simulink model "Solar_panel"  (R2024a)
settings: Solver=VariableStepAuto  StartTime=0.0  StopTime=1000  RelTol=1e-3
libraries: ee_lib x36, fl_lib x5, nesl_utility x4, simulink x1
settings Model: SimulationMode=accelerator  Creator=glenn  LastModifiedBy=glenn

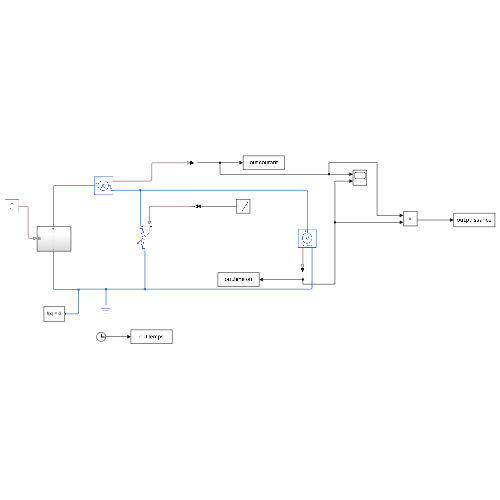
[thumbnail: Simulink's stored preview of the top-level diagram]
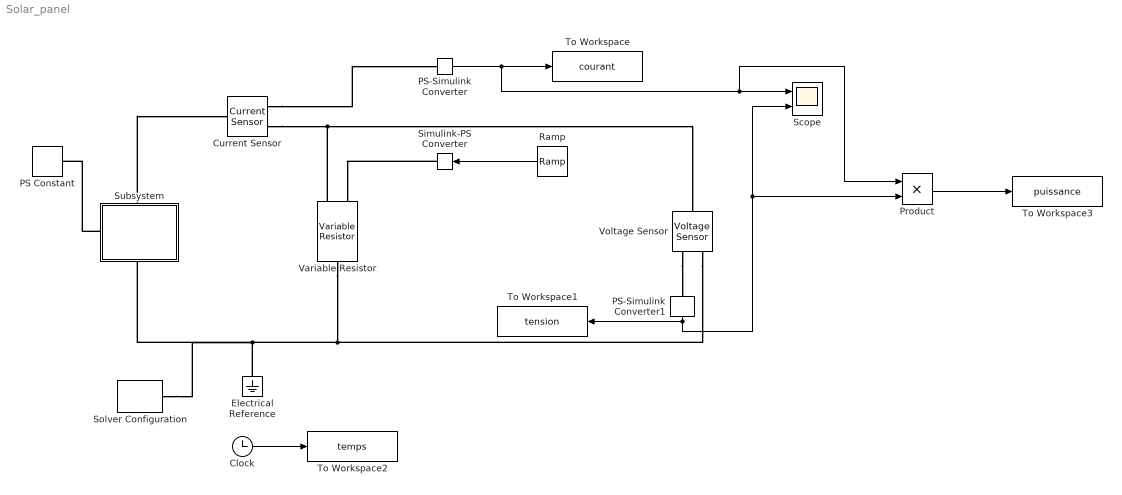
== system Solar_panel ==
  Clock : Clock
  Current Sensor : fl_lib/Electrical/Electrical Sensors/Current Sensor
  Electrical Reference : fl_lib/Electrical/Electrical Elements/Electrical Reference
  PS Constant : fl_lib/Physical Signals/Sources/PS Constant  constant=1000
  PS-Simulink Converter : nesl_utility/PS-Simulink Converter  PhysicalDomain=network_engine_domain  SubClassName=ps_output  LeftPortType=input  RightPortType=output  PseudoPeriodic=off  Frequencies=[]  VectorFormat=inherit  Unit=inherit  AffineConversion=off
  PS-Simulink Converter1 : nesl_utility/PS-Simulink Converter  PhysicalDomain=network_engine_domain  SubClassName=ps_output  LeftPortType=input  RightPortType=output  PseudoPeriodic=off  Frequencies=[]  VectorFormat=inherit  Unit=inherit  AffineConversion=off
  Product : Product
  Ramp : simulink/Sources/Ramp  slope=1  start=0  InitialOutput=0
  Scope : Scope  NumInputPorts=2
  Simulink-PS Converter : nesl_utility/Simulink-PS Converter  PhysicalDomain=network_engine_domain  SubClassName=ps_input  LeftPortType=input  RightPortType=output  PseudoPeriodic=off  Frequencies=[]  NoiseDistribution=none  NoiseParameters=[]  Unit=1  AffineConversion=off  FilteringAndDerivatives=provide  SimscapeFilterOrder=1  InputFilterTimeConstant=0.001  UdotUserProvided=0
  Solver Configuration : nesl_utility/Solver Configuration  PhysicalDomain=network_engine_domain  SubClassName=solver  LeftPortType=input  RightPortType=generic  Tones=[]  Harmonics=[]  SimulateNoise=off  Profile=off  UseLocalSampling=off  EnableSwitchedLinearOptims=on  FrequencyDomain=off  UseCCode=off  RelTol=0.001  AbsTol=0.001  MinStep=1e-09  ToWorkspace=off  RevertToSquareIcSolve=off  NumHomotopyIterations=100  PhasorMode=off  PhasorModeNumHarmonics=1  ConsistencySolver=NEWTON_XTOL_AFTER_FTOL  IndexReductionMethod=DerivativeReplacement  DoDC=off  ResidualTolerance=1e-09  ConsistencyTolSource=GLOBAL  ConsistencyAbsTol=0.001  ConsistencyRelTol=0.001  ConsistencyTolFactor=1e-9  UseLocalSolver=on  LocalSolverChoice=NE_BACKWARD_EULER_ADVANCER  ResolveIndetEquations=on  FunctionEvalNumThread=1  LocalSolverSampleTime=0.001  DoFixedCost=on  MaxNonlinIter=3  MaxModeIter=2  ComputeImpulses=off  ImpulseIterations=2  LinearAlgebra=auto  LinearAlgebraNumThread=0  EquationFormulation=NE_TIME_EF  DelaysMemoryBudget=1024  AutomaticFiltering=on  FilteringTimeConstant=0.001  PartitionStorageMethod=AS_NEEDED  PartitionMemoryBudget=1024  PartitionMethod=ROBUST  MultibodyUseLocalSolver=off  MultibodyLocalSolverChoice=ODE1  MultibodyLocalSolverSampleTime=0.001
  Subsystem : Subsystem
      settings: PortSchema="{\"entries\":[{\"content\":{\"sides\":[{\"content\":{},\"type\":\"ConnectorPlacement.EquallySpacedRectSide\",\"uuid\":\"4a140c86-2c53-43bf-a36e-a1c263b6c553\"},{\"content\":{\"connectorIds\":[\"RConn1\"],\"side\":\"RIGHT\"},\"type\":\"ConnectorPlacement.EquallySpacedRectSide\",\"uuid\":\"ded2075e-c008-496e-9eaf-35fc0cc51be6\"},{\"content\":{\"connectorIds\":[\"LConn1\"],\"side\":\"TOP\"},\"type\":\"ConnectorPlacement.EquallySpacedRectSide\",\"uuid\":\"5598b79a-9572-4b58-9bc6-3a372ecc07ee\"},{\"content\":{\"connectorIds\":[\"RConn2\"],\"side\":\"BOTTOM\"},\"type\":\"ConnectorPlacement.EquallySpacedRectSide\",\"uuid\":\"8596b7d6-c7dc-49d4-be1e-6b0e22e75e30\"}]},\"type\":\"ConnectorPlacement.EquallySpacedConnector\",\"uuid\":\"cc072fb6-9e77-4cb7-a941-2671d66ee608\"}],\"packageUris\":[\"http://schema.mathworks.com/mf0/Connector/R2020b\"],\"version\":\"1.0\"}"
  To Workspace : ToWorkspace  VariableName=courant  SampleTime=-1
  To Workspace1 : ToWorkspace  VariableName=tension  SampleTime=-1
  To Workspace2 : ToWorkspace  VariableName=temps  SaveFormat=Timeseries  SampleTime=-1
  To Workspace3 : ToWorkspace  VariableName=puissance  SampleTime=-1
  Variable Resistor : fl_lib/Electrical/Electrical Elements/Variable Resistor  Rmin=0 Ohm  thermalEnable=false  thermal_mass=1 J/K  i_specify=off  i_priority=None  i=0 A  i_nominal_specify=off  i_nominal_value=1  i_nominal_unit=A  v_specify=off  v_priority=None  v=0 V  v_nominal_specify=off  v_nominal_value=1  v_nominal_unit=V  T_specify=off  T_priority=None  T=300 K  T_nominal_specify=off  T_nominal_value=1  T_nominal_unit=K
  Voltage Sensor : fl_lib/Electrical/Electrical Sensors/Voltage Sensor
  wires:
  PS-Simulink Converter/1 -> Product/1, Scope/1, To Workspace/1
  PS-Simulink Converter1/1 -> To Workspace1/1, Product/2, Scope/2
  Clock/1 -> To Workspace2/1
  Ramp/1 -> Simulink-PS Converter/1
  Product/1 -> To Workspace3/1
  connections:
  Current Sensor/RConn2 -- Variable Resistor/LConn2 -- Voltage Sensor/LConn1
  Voltage Sensor/RConn2 -- Variable Resistor/RConn1 -- Subsystem/RConn2 -- Solver Configuration/RConn1 -- Electrical Reference/LConn1
  Current Sensor/RConn1 -- PS-Simulink Converter/LConn1
  Voltage Sensor/RConn1 -- PS-Simulink Converter1/LConn1
  Simulink-PS Converter/RConn1 -- Variable Resistor/LConn1
  Subsystem/RConn1 -- PS Constant/RConn1
  Subsystem/LConn1 -- Current Sensor/LConn1

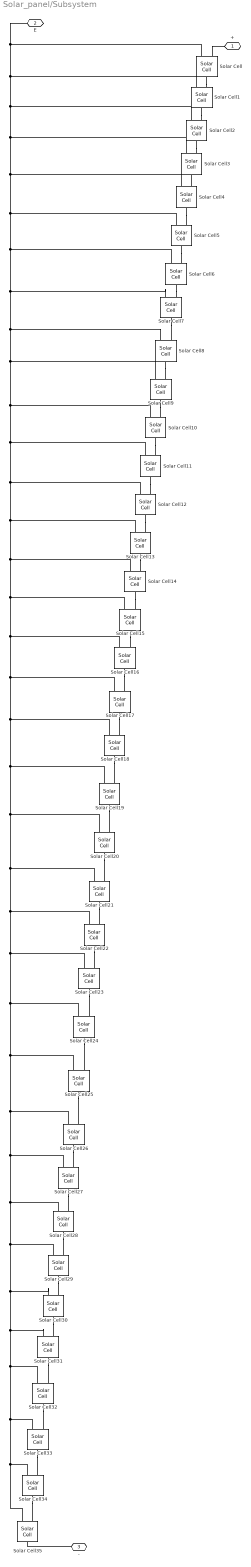
== system Solar_panel/Subsystem ==
  Solar Cell : ee_lib/Sources/Solar Cell  prm=1  Isc=0.30 A  Voc=0.62 V  Is=1e-6 A  Is2=0 A  Iph=7.34 A  Ir0=1000 W/m^2  ec=1.5  N2=2  Rs=0 Ohm  Rp=inf Ohm  N_series=1  N_parallel=1  TIPH1=0 1/K  EG=1.11 eV  TXIS1=3  TXIS2=3  TRS1=0  TRP1=0  Tmeas=25 degC  TFIXED=25 degC  thermal_mass=100 J/K  initial_temperature=25 degC
  Solar Cell{1..35} (35 alike) : ee_lib/Sources/Solar Cell  prm=1  Isc=0.3 A  Voc=0.62 V  Is=1e-6 A  Is2=0 A  Iph=7.34 A  Ir0=1000 W/m^2  ec=1.5  N2=2  Rs=0 Ohm  Rp=inf Ohm  N_series=1  N_parallel=1  TIPH1=0 1/K  EG=1.11 eV  TXIS1=3  TXIS2=3  TRS1=0  TRP1=0  Tmeas=25 degC  TFIXED=25 degC  thermal_mass=100 J/K  initial_temperature=25 degC
  + : PMIOPort  Side=Left
  E : PMIOPort  Port=2  Side=Right
  - : PMIOPort  Port=3  Side=Right
  connections:
  Solar Cell1/LConn1 -- Solar Cell/LConn1 -- E/RConn1 -- Solar Cell2/LConn1 -- Solar Cell3/LConn1 -- Solar Cell4/LConn1 -- Solar Cell5/LConn1 -- Solar Cell6/LConn1 -- Solar Cell7/LConn1 -- Solar Cell30/LConn1 -- Solar Cell31/LConn1 -- Solar Cell32/LConn1 -- Solar Cell33/LConn1 -- Solar Cell34/LConn1 -- Solar Cell35/LConn1 -- Solar Cell29/LConn1 -- Solar Cell28/LConn1 -- Solar Cell27/LConn1 -- Solar Cell26/LConn1 -- Solar Cell25/LConn1 -- Solar Cell24/LConn1 -- Solar Cell23/LConn1 -- Solar Cell22/LConn1 -- Solar Cell21/LConn1 -- Solar Cell20/LConn1 -- Solar Cell19/LConn1 -- Solar Cell18/LConn1 -- Solar Cell17/LConn1 -- Solar Cell16/LConn1 -- Solar Cell15/LConn1 -- Solar Cell14/LConn1 -- Solar Cell13/LConn1 -- Solar Cell12/LConn1 -- Solar Cell11/LConn1 -- Solar Cell10/LConn1 -- Solar Cell9/LConn1 -- Solar Cell8/LConn1
  +/RConn1 -- Solar Cell/LConn2
  Solar Cell/RConn1 -- Solar Cell1/LConn2
  Solar Cell1/RConn1 -- Solar Cell2/LConn2
  Solar Cell2/RConn1 -- Solar Cell3/LConn2
  Solar Cell4/LConn2 -- Solar Cell3/RConn1
  Solar Cell4/RConn1 -- Solar Cell5/LConn2
  Solar Cell5/RConn1 -- Solar Cell6/LConn2
  Solar Cell6/RConn1 -- Solar Cell7/LConn2
  Solar Cell7/RConn1 -- Solar Cell8/LConn2
  Solar Cell8/RConn1 -- Solar Cell9/LConn2
  Solar Cell9/RConn1 -- Solar Cell10/LConn2
  Solar Cell10/RConn1 -- Solar Cell11/LConn2
  Solar Cell11/RConn1 -- Solar Cell12/LConn2
  Solar Cell12/RConn1 -- Solar Cell13/LConn2
  Solar Cell13/RConn1 -- Solar Cell14/LConn2
  Solar Cell14/RConn1 -- Solar Cell15/LConn2
  Solar Cell15/RConn1 -- Solar Cell16/LConn2
  Solar Cell16/RConn1 -- Solar Cell17/LConn2
  Solar Cell17/RConn1 -- Solar Cell18/LConn2
  Solar Cell18/RConn1 -- Solar Cell19/LConn2
  Solar Cell19/RConn1 -- Solar Cell20/LConn2
  Solar Cell20/RConn1 -- Solar Cell21/LConn2
  Solar Cell21/RConn1 -- Solar Cell22/LConn2
  Solar Cell22/RConn1 -- Solar Cell23/LConn2
  Solar Cell23/RConn1 -- Solar Cell24/LConn2
  Solar Cell24/RConn1 -- Solar Cell25/LConn2
  Solar Cell25/RConn1 -- Solar Cell26/LConn2
  Solar Cell26/RConn1 -- Solar Cell27/LConn2
  Solar Cell27/RConn1 -- Solar Cell28/LConn2
  Solar Cell28/RConn1 -- Solar Cell29/LConn2
  Solar Cell29/RConn1 -- Solar Cell30/LConn2
  Solar Cell30/RConn1 -- Solar Cell31/LConn2
  Solar Cell31/RConn1 -- Solar Cell32/LConn2
  Solar Cell32/RConn1 -- Solar Cell33/LConn2
  Solar Cell33/RConn1 -- Solar Cell34/LConn2
  Solar Cell34/RConn1 -- Solar Cell35/LConn2
  -/RConn1 -- Solar Cell35/RConn1
